simulink model "TRN_V3_2_CodeGen"  (R2022a)
settings: Solver=FixedStepAuto  StartTime=0.0  StopTime=300  FixedStep=0.04  RelTol=1e-3
PreLoadFcn:
  | load('BusStructureTRNsensor.mat');
  | addpath('C:/MAP');
InitFcn:
  | %load TRNDataBusPILS.mat
  | %addpath(genpath(cd))
  | 
  | %load('TPF_WHOLESIM_INPUT_SCENARIOS_AGCAS_N35_10E127_70.mat');
  | 
  | % Add DataBus Path
  | addpath(',,/');
  | addpath('../MAP/');
  | addpath('../MAP/MAP_DB');
  | addpath('../MAP/DVOF');
  | addpath(genpath(cd));
  | load('BusStructureTRN.mat');
undefined symbols (not defined in the file or in its folder): Altitude_INS, Latitude_INS, Longitude_INS, TRN, TRNlib
libraries: simulink_extras x23, aerolibconvert2 x6, sharedtransform x4, dspstat3 x2
(part 1 of 3)
settings Model: Creator=HSU  LastModifiedBy=ASCL
settings OptimizationCC: DefaultParameterBehavior=Inlined  UseDivisionForNetSlopeComputation=on  GainParamInheritBuiltInType=on  UseFloatMulNetSlope=on  PassReuseOutputArgsAs=Individual arguments  ZeroExternalMemoryAtStartup=off  ZeroInternalMemoryAtStartup=off  LifeSpan=Inf  OptimizeBlockOrder=speed  DifferentSizesBufferReuse=on  EfficientTunableParamExpr=on
settings DebuggingCC: ParameterTunabilityLossMsg=error  UnconnectedInputMsg=warning  UnconnectedOutputMsg=warning  UnconnectedLineMsg=warning  SFUnexpectedBacktrackingDiag=warning  SFNoUnconditionalDefaultTransitionDiag=warning
settings HardwareCC: ProdBitPerPointer=32  ProdBitPerSizeT=32  ProdBitPerPtrDiffT=32  ProdLargestAtomicInteger=Long  ProdLargestAtomicFloat=Double  ProdEndianess=BigEndian  ProdWordSize=32  ProdLongLongMode=on  ProdHWDeviceType=Freescale->MPC83xx
settings ModelReferenceCC: ModelReferenceNumInstancesAllowed=Single
settings SFSimCC: SimCustomHeaderCode="#include \"MAP.h\""  SimUserSources=MAP.c  SimUserLibraries=WS2_32.LIB  MATLABDynamicMemAlloc=off
settings RTWCC: SystemTargetFile=ert.tlc  GenCodeOnly=on  TemplateMakefile=ert_default_tmf  GenerateReport=on  RTWUseSimCustomCode=on  CustomHeaderCode="#include \"MAP.h\""  CustomSource=MAP.c  CustomLibrary=WS2_32.LIB  BuildConfiguration=Faster Runs  LaunchReport=on  GenerateCodeMetricsReport=on  DLArmComputeVersion=19.05
settings CodeAppCC: ForceParamTrailComments=on  IgnoreCustomStorageClasses=off  OperatorAnnotations=on  SimulinkDataObjDesc=on  SFDataObjDesc=on  MATLABFcnDesc=on  InsertBlockDesc=on  StateflowObjectComments=on  MATLABSourceComments=on  EnableCustomComments=on  ReqsInCode=on
settings ERTTargetCC: TargetLangStandard=C99 (ISO)  UtilityFuncGeneration=Shared location  GenerateSampleERTMain=on  SuppressErrorStatus=on  SupportAbsoluteTime=off  SupportNonFinite=off  SupportComplex=off  SupportVariableSizeSignals=on  ParenthesesLevel=Standards  CastingMode=Standards  InlinedParameterPlacement=NonHierarchical  ERTCustomFileTemplate=example_file_process.tlc  PreserveIfCondition=on  ConvertIfToSwitch=off  EnableSignedLeftShifts=off  EnableSignedRightShifts=off

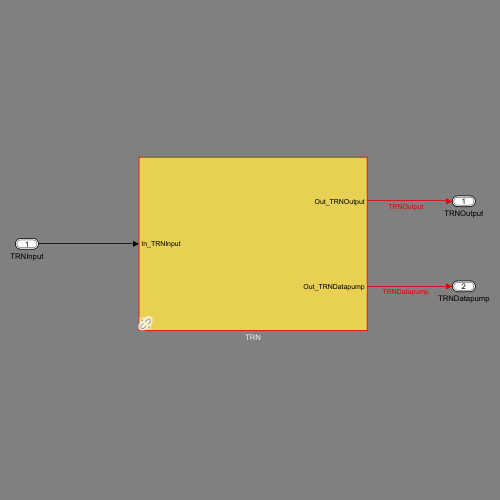
[thumbnail: Simulink's stored preview of the top-level diagram]
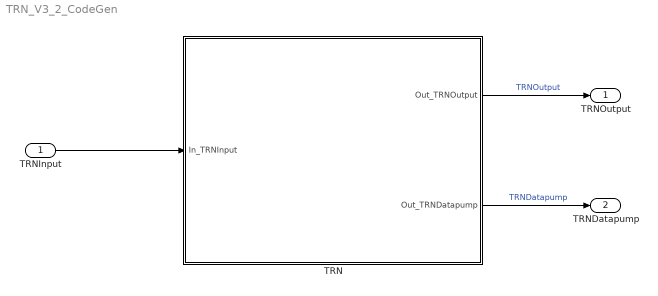
== system TRN_V3_2_CodeGen ==
  TRNInput : Inport  OutDataTypeStr=Bus: TRNInput  BusOutputAsStruct=on
  TRN : Subsystem  AncestorBlock=TRNlib/TRN
  TRNOutput : Outport  OutDataTypeStr=Bus: TRNOutput  VectorParamsAs1DForOutWhenUnconnected=off  BusOutputAsStruct=on
  TRNDatapump : Outport  Port=2  OutDataTypeStr=Bus: TRNDatapump  VectorParamsAs1DForOutWhenUnconnected=off  BusOutputAsStruct=on
  wires:
  TRN/2(Out_TRNDatapump) -> TRNDatapump/1  "TRNDatapump"
  TRN/1(Out_TRNOutput) -> TRNOutput/1  "TRNOutput"
  TRNInput/1 -> TRN/1(In_TRNInput)

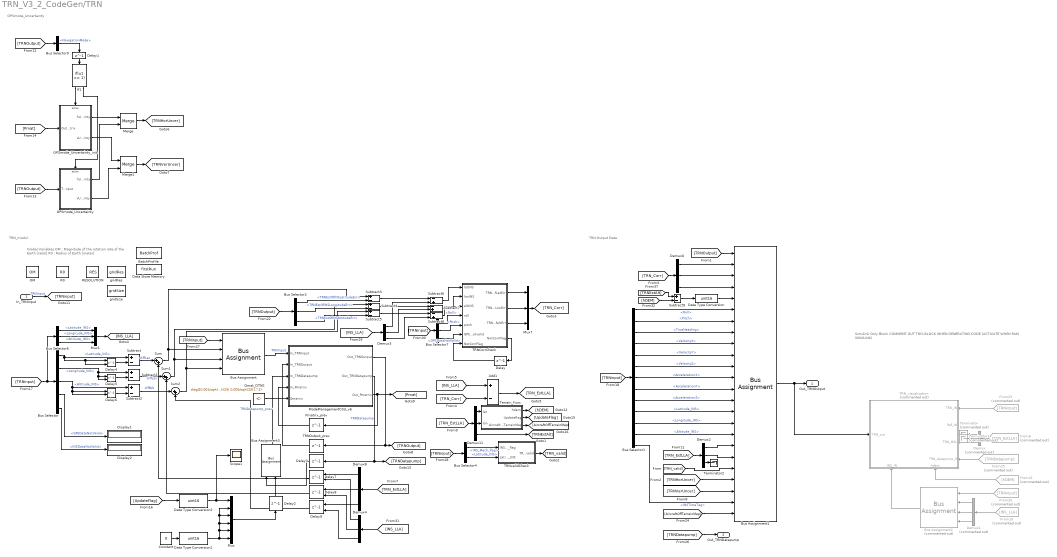
== system TRN_V3_2_CodeGen/TRN ==
  note: Global Variables
      | OM : Magnitude of the rotation rate of the Earth [rad/s]
      | R0 : Radius of Earth [meter]
  note: GPSmode_Uncertainty
  note: TRN Output Data
  note: TRN_modul
  note: Simulink Only Block
      | COMMENT OUT THIS BLOCK WHEN GENERATING CODE
      | (ACTIVATE WHEN RUN SIMULINK)
  In_TRNInput : Inport  OutDataTypeStr=Bus: TRNInput
  Add1 : Sum  Inputs=+-
  BatchProfile : DataStoreMemory  DataStoreName=BatchProf  ReadBeforeWriteMsg=warning  WriteAfterWriteMsg=warning  WriteAfterReadMsg=warning  ShowAdditionalParam=off  OutDataTypeStr=double  Dimensions=84200
  Bus Assignment : BusAssignment  AssignedSignals=Latitude_INS,Longitude_INS,Altitude_INS
  Bus Assignment1 : BusAssignment  AssignedSignals=TRNEstOfINSLatitudeErr,TRNEstOfINSLongitudeErr,TRNEstOfINSAltitudeErr,TRNEstHeightAGL,TRN_Roll,TRN_Pitch,TRN_Yaw,TRN_VelocityX,TRN_VelocityY,TRN_VelocityZ,TRN_AccelerationX,TRN_AccelerationY,TRN_AccelerationZ,Latitude_INS,Longitude_INS,Altitude_INS,TRNEstOfLatitude,TRNEstOfLongitude,TRN_valid,TRNHorUncertainty,TRNVerticalUncertainty,TRNTimeTag,AircraftOffTerrainMap
  Bus Assignment2 : BusAssignment  Commented=on  AssignedSignals=Latitude_INS,Longitude_INS,Altitude_INS
  Bus Assignment3 : BusAssignment  AssignedSignals=Result_Prev
  Bus Selector : BusSelector  OutputSignals=Latitude_INS,Longitude_INS,Altitude_INS,GPSDataNotValid,INSDataNotValid
  Bus Selector1 : BusSelector  OutputSignals=Roll,Pitch,TrueHeading,VelocityX,VelocityY,VelocityZ,AccelerationX,AccelerationY,AccelerationZ,Latitude_INS,Longitude_INS,Altitude_INS,INSTimeTag
  Bus Selector2 : BusSelector  OutputSignals=TRNEstOfINSLatitudeErr,TRNEstOfINSLongitudeErr,TRNEstOfINSAltitudeErr
  Bus Selector4 : BusSelector  OutputSignals=INS_Mech_flag,Latitude_INS
  Bus Selector6 : BusSelector  OutputSignals=Latitude_INS,Longitude_INS,Altitude_INS
  Bus Selector7 : BusSelector  OutputSignals=Roll,Pitch,GPSDataNotValid
  Bus Selector9 : BusSelector  OutputSignals=NavigationMode
  Constant : Constant  Value=0
  Data Store Memory : DataStoreMemory  DataStoreName=firstRun  ReadBeforeWriteMsg=warning  WriteAfterWriteMsg=warning  WriteAfterReadMsg=warning  InitialValue=logical(1)  VectorParams1D=off  ShowAdditionalParam=off  OutDataTypeStr=boolean
      settings: LockScale=on
  Data Type Conversion : DataTypeConversion  OutDataTypeStr=uint16  RndMeth=Nearest  SaturateOnIntegerOverflow=off
  Data Type Conversion1 : DataTypeConversion  OutDataTypeStr=uint16  SaturateOnIntegerOverflow=off  RndMeth=Floor
  Data Type Conversion2 : DataTypeConversion  OutDataTypeStr=uint16  SaturateOnIntegerOverflow=off  RndMeth=Floor
  Delay : Delay  DelayLength=1
  Delay1 : Delay  DelayLength=1  InitialCondition=1
  Delay2 : Delay  DelayLength=1  InitialCondition=0
  Delay3 : Delay  DelayLength=1  InitialCondition=0
  Delay4 : Delay  DelayLength=1  InitialConditionSource=Input port  InitialCondition=35.2*pi/180
      settings: InputPortMap=u0,p4
  Delay5 : Delay  DelayLength=1  InitialConditionSource=Input port  InitialCondition=35.2*pi/180
      settings: InputPortMap=u0,p4
  Delay6 : Delay  DelayLength=1  InitialConditionSource=Input port  InitialCondition=35.2*pi/180
      settings: InputPortMap=u0,p4
  Delay7 : Delay  DelayLength=1  InitialConditionSource=Input port  InitialCondition=0
      settings: InputPortMap=u0,p4
  Delay8 : Delay  DelayLength=1  InitialConditionSource=Input port  InitialCondition=0
      settings: InputPortMap=u0,p4
  Delay9 : Delay  DelayLength=1  InitialConditionSource=Input port  InitialCondition=0
      settings: InputPortMap=u0,p4
  Demux : Demux  Commented=on  Outputs=3
  Demux1 : Demux  Commented=on  Outputs=3
  Demux{2..4,6,8,11} (6 alike) : Demux  Outputs=3
  Display1 : Display
  Display2 : Display
  From10 : From  Commented=on  GotoTag=INS_LLA
  From20 : From  Commented=on  GotoTag=TRNinput
  From21 : From  Commented=on  GotoTag=hDEM
  From23 : From  Commented=on  GotoTag=TRNinput
  From25 : From  Commented=on  GotoTag=TRNDatapump
  From6 : From  Commented=on  GotoTag=TRN_EstLLA
  GPSmode_Uncertainty : Subsystem  TreatAsAtomicUnit=on
  GPSmode_Uncertainty_init : Subsystem  TreatAsAtomicUnit=on
  If1 : If  IfExpression=u1 == 1
  Merge : Merge
  Merge1 : Merge
  ModeManagementCSU_v6 : Stateflow chart  TreatAsAtomicUnit=on
  Mux : Mux  Inputs=6
  Mux1 : Mux  Inputs=3
  Mux7 : Mux  Inputs=3
  OM : DataStoreMemory  DataStoreName=OM  ReadBeforeWriteMsg=warning  WriteAfterWriteMsg=warning  WriteAfterReadMsg=warning  InitialValue=7.27e-5  ShowAdditionalParam=off
  Pmatrix_prev : Delay  DelayLength=1  InitialCondition="diag([0 0 0 0 0 0  10/6378000 10/6378000 13.3 0.0 0.0 0.0 0.00014 0.00014 0.00014 ].^2);"
  Qmat_DTNS : Constant  Value=diag([0.001/sqrt(25) 0.001/sqrt(25) 0.001/sqrt(25) 0.005/sqrt(25) 0.005/sqrt(25) 0.005/sqrt(25)].^2)
  R0 : DataStoreMemory  DataStoreName=R0  ReadBeforeWriteMsg=warning  WriteAfterWriteMsg=warning  WriteAfterReadMsg=warning  InitialValue=6378000  ShowAdditionalParam=off
  RESOLUTION : DataStoreMemory  DataStoreName=RES  ReadBeforeWriteMsg=warning  WriteAfterWriteMsg=warning  WriteAfterReadMsg=warning  InitialValue=3 * 0.000277777777777777 * 0.0174532925199433  ShowAdditionalParam=off  OutDataTypeStr=double
  Scope1 : Scope
  Subtract{,1..5,9} (7 alike) : Sum  Inputs=+-
  Subtract6 : Sum  Inputs=-+
  Subtract7 : Sum  Inputs=-+
  Subtract8 : Sum  Inputs=-+
  Sum : Sum  Inputs=|++
  Sum1 : Sum  Inputs=|++
  Sum2 : Sum  Inputs=|++
  TRNCorrCheck : MATLAB Function  TreatAsAtomicUnit=on
  TRNOutput_prev : Delay  DelayLength=1  InitialCondition=struct('NavigationMode', false);
  "TRN_visualization " : Subsystem  Commented=on
      settings: PortSchema="{\"entries\":[{\"content\":{\"sides\":[{\"content\":{\"connectorIds\":[\"In1\",\"In2\",\"In3\",\"In4\"]},\"type\":\"ConnectorPlacement.EquallySpacedRectSide\",\"uuid\":\"9b00cbc4-ca0d-429d-9536-38963fe71bc1\"},{\"content\":{\"connectorIds\":[\"In7\"],\"side\":\"RIGHT\"},\"type\":\"ConnectorPlacement.EquallySpacedRectSide\",\"uuid\":\"1db309fb-4b82-499a-a8dc-4a1ba85275fb\"},{\"content\":{\"connectorIds\":[\"In5\",\"In6\"],\"side\":\"TOP\"},\"type\":\"ConnectorPlacement.EquallySpacedRectSide\",\"uuid\":\"7e2d2316-30f0-423f-b46b-636ee0f4a770\"}]},\"type\":\"ConnectorPlacement.EquallySpacedConnector\",\"uuid\":\"aa6e905d-ed4c-45ad-a850-3c33939aad22\"}],\"packageUris\":[\"http://schema.mathworks.com/mf0/Connector/R2020b\"],\"version\":\"1.0\"}"
  TRNvalidCheck : MATLAB Function  TreatAsAtomicUnit=on
  Terminator : Terminator  Commented=on
  Terminator1 : Terminator  Commented=on
  Terminator2 : Terminator
  Terrain_Func : Subsystem
  gridRes : DataStoreMemory  DataStoreName=gridRes  ReadBeforeWriteMsg=warning  WriteAfterWriteMsg=warning  WriteAfterReadMsg=warning  InitialValue=0.1  ShowAdditionalParam=off  OutDataTypeStr=double
  gridSize : DataStoreMemory  DataStoreName=gridSize  ReadBeforeWriteMsg=warning  WriteAfterWriteMsg=warning  WriteAfterReadMsg=warning  InitialValue=20  ShowAdditionalParam=off  OutDataTypeStr=double
  Out_TRNOutput : Outport  OutDataTypeStr=Bus: TRNOutput  VectorParamsAs1DForOutWhenUnconnected=off
  Out_TRNDatapump : Outport  Port=2  OutDataTypeStr=Bus: TRNDatapump  VectorParamsAs1DForOutWhenUnconnected=off
  wires:
  Bus Selector2/2 -> Subtract4/2  "<TRNEstOfINSLongitudeErr>"
  Bus Selector2/1 -> Subtract3/2  "<TRNEstOfINSLatitudeErr>"
  Terrain_Func/1(hdem) -> [hDEM]
  Bus Selector4/1 -> TRNvalidCheck/1(INS_Mech_flag)  "<INS_Mech_flag>"
  Bus Selector4/2 -> TRNvalidCheck/2(Latitude_INS)  "<Latitude_INS>"
  [TRN_valid] -> Bus Assignment1/20
  TRNvalidCheck/1(TRN_valid) -> [TRN_valid]
  Bus Assignment/1 -> ModeManagementCSU_v6/1(In_TRNInput)  "TRNInput"
  Bus Selector/2 -> Delay5/1, Delay5/2, Subtract1/1  "<Longitude_INS>"
  Bus Selector1/3 -> Bus Assignment1/8  "<TrueHeading>"
  Bus Selector1/12 -> Bus Assignment1/17  "<Altitude_INS>"
  Bus Selector1/11 -> Bus Assignment1/16  "<Longitude_INS>"
  Bus Selector1/10 -> Bus Assignment1/15  "<Latitude_INS>"
  Bus Selector1/9 -> Bus Assignment1/14  "<AccelerationZ>"
  Bus Selector1/8 -> Bus Assignment1/13  "<AccelerationY>"
  Bus Selector1/7 -> Bus Assignment1/12  "<AccelerationX>"
  Bus Selector1/6 -> Bus Assignment1/11  "<VelocityZ>"
  Bus Selector1/5 -> Bus Assignment1/10  "<VelocityY>"
  Bus Selector1/4 -> Bus Assignment1/9  "<VelocityX>"
  Bus Selector1/2 -> Bus Assignment1/7  "<Pitch>"
  Bus Selector1/1 -> Bus Assignment1/6  "<Roll>"
  In_TRNInput/1 -> [TRNinput]  "TRNInput"
  ModeManagementCSU_v6/2(Out_TRNDatapump) -> Delay3/1, [TRNDatapump]  "TRNDatapump"
  TRNOutput_prev/1 -> ModeManagementCSU_v6/2(In_TRNOutput)
  Delay3/1 -> Bus Assignment3/1
  Bus Selector/3 -> Delay6/2, Delay6/1, Subtract2/1  "<Altitude_INS>"
  Bus Selector/1 -> Delay4/1, Delay4/2, Subtract/1  "<Latitude_INS>"
  Delay4/1 -> Subtract/2
  Delay5/1 -> Subtract1/2
  Delay6/1 -> Subtract2/2
  Sum/1 -> Subtract3/1, Bus Assignment/2
  Sum1/1 -> Subtract4/1, Bus Assignment/3
  Sum2/1 -> Subtract5/1, Bus Assignment/4
  Subtract/1 -> Sum/1  "diffLat"
  Subtract1/1 -> Sum1/1  "diffLon"
  Subtract4/1 -> Subtract7/1
  Subtract2/1 -> Sum2/1  "diffAlt"
  Delay7/1 -> Sum/2
  Delay8/1 -> Sum1/2
  Delay9/1 -> Sum2/2
  Bus Assignment1/1 -> "TRN_visualization "/7(TRN_out), Out_TRNOutput/1
  Subtract9/1 -> Data Type Conversion/1
  Data Type Conversion/1 -> Bus Assignment1/5
  Subtract6/1 -> TRNCorrCheck/1(latINS)
  Subtract7/1 -> TRNCorrCheck/2(lonINS)
  Subtract8/1 -> TRNCorrCheck/3(altINS)
  TRNCorrCheck/3(TRNEstOfaltErr) -> Mux7/3
  [TRN_Corr] -> Demux6/1
  Demux6/1 -> Bus Assignment1/2
  Demux6/2 -> Bus Assignment1/3
  Demux6/3 -> Bus Assignment1/4
  TRNCorrCheck/1(TRNEstOfLatErr) -> Mux7/1
  TRNCorrCheck/2(TRNEstOfLonErr) -> Mux7/2
  Subtract5/1 -> Subtract8/1
  Subtract3/1 -> Subtract6/1
  [TRN_EstLLA] -> Demux8/1
  Demux8/1 -> Delay7/1
  Demux8/2 -> Delay8/1
  Demux8/3 -> Delay9/1
  Mux1/1 -> [INS_LLA]
  Bus Selector6/2 -> Mux1/2  "<Longitude_INS>"
  Bus Selector6/3 -> Mux1/3  "<Altitude_INS>"
  [INS_LLA] -> Add1/1
  Add1/1 -> [TRN_EstLLA]
  Demux11/1 -> Terrain_Func/1(lat)
  Demux11/2 -> Terrain_Func/2(lon)
  TRNCorrCheck/4(NotCorrFlag) -> Delay/1
  Delay/1 -> TRNCorrCheck/7("NotCorrFlag ")
  [TRN_EstLLA] -> Demux11/1
  Qmat_DTNS/1 -> ModeManagementCSU_v6/5(Qmatrix)
  ModeManagementCSU_v6/3(Out_Pmatrix) -> Pmatrix_prev/1, [Pmat]
  Bus Selector/4 -> Display1/1  "<GPSDataNotValid>"
  Mux7/1 -> [TRN_Corr]
  If1/1 -> GPSmode_Uncertainty_init/Action
  If1/2 -> GPSmode_Uncertainty/Action
  GPSmode_Uncertainty_init/1(hUncertainty) -> Merge/1
  GPSmode_Uncertainty/1(hUncertainty) -> Merge/2
  GPSmode_Uncertainty_init/2(vUncertainty) -> Merge1/1
  GPSmode_Uncertainty/2(vUncertainty) -> Merge1/2
  Bus Selector9/1 -> Delay1/1  "<NavigationMode>"
  Merge/1 -> [TRNHorUncer]
  Merge1/1 -> [TRNVerUncer]
  [TRNVerUncer] -> Bus Assignment1/22
  Demux2/1 -> Bus Assignment1/18
  Demux2/2 -> Bus Assignment1/19
  [TRN_EstLLA] -> Demux2/1
  [TRNOutput] -> Bus Selector9/1
  [TRNOutput] -> GPSmode_Uncertainty/1(TRNOutput)
  [Pmat] -> GPSmode_Uncertainty_init/1(Out_Pmatrix)
  [TRNinput] -> Bus Selector6/1, Bus Selector/1
  [TRNinput] -> Bus Selector1/1
  [TRNDatapump] -> Out_TRNDatapump/1
  [TRNinput] -> Bus Assignment/1
  Delay1/1 -> If1/1
  [TRNOutput] -> Bus Assignment1/1
  Bus Selector2/3 -> Subtract5/2  "<TRNEstOfINSAltitudeErr>"
  [TRNOutput] -> Bus Selector2/1
  [INS_LLA] -> Demux3/1
  Demux3/1 -> Subtract6/2
  Demux3/2 -> Subtract7/2
  Demux3/3 -> Subtract8/2
  [TRNinput] -> Bus Selector7/1
  Bus Selector7/1 -> TRNCorrCheck/4(roll)  "<Roll>"
  Bus Selector7/2 -> TRNCorrCheck/5(pitch)  "<Pitch>"
  Bus Selector6/1 -> Mux1/1  "<Latitude_INS>"
  [INS_LLA] -> Demux4/1
  Demux4/1 -> Delay7/2
  Demux4/2 -> Delay8/2
  Demux4/3 -> Delay9/2
  Bus Selector7/3 -> TRNCorrCheck/6(GPSDataNotvalid)  "<GPSDataNotValid>"
  [hDEM] -> Subtract9/2
  Demux11/3 -> [TRNEstAlt]
  [TRNEstAlt] -> Subtract9/1
  Bus Selector1/13 -> Bus Assignment1/23  "<INSTimeTag>"
  Bus Assignment2/1 -> "TRN_visualization "/6(INS_IN)
  Demux1/1 -> Bus Assignment2/2
  From20/1 -> Bus Assignment2/1
  From10/1 -> Demux1/1
  From6/1 -> Demux/1
  From23/1 -> "TRN_visualization "/4(TRN_IN)
  Demux/3 -> "TRN_visualization "/2(TRN_MSL)
  From21/1 -> "TRN_visualization "/5(hdem)
  Demux1/3 -> Bus Assignment2/4
  From25/1 -> "TRN_visualization "/1(TRN_datapump_IN)
  Demux1/2 -> Bus Assignment2/3
  Bus Assignment3/1 -> ModeManagementCSU_v6/3(In_TRNDatapump)  "TRNDatapump_prev"
  [TRNinput] -> Bus Selector4/1
  ModeManagementCSU_v6/1(Out_TRNOutput) -> TRNOutput_prev/1, [TRNOutput]
  [TRNHorUncer] -> Bus Assignment1/21
  Bus Selector/5 -> Display2/1  "<INSDataNotValid>"
  [TRN_Corr] -> Add1/2
  Mux/1 -> Delay2/1
  Terrain_Func/2(Updateflag) -> [UpdateFlag]
  Constant/1 -> Data Type Conversion1/1
  Terrain_Func/3(AircraftOffTerrainMap) -> [AircraftOffTerrainMap]
  [AircraftOffTerrainMap] -> Bus Assignment1/24
  Data Type Conversion1/1 -> Mux/2, Mux/3, Mux/4, Mux/5, Mux/6
  [UpdateFlag] -> Data Type Conversion2/1
  Data Type Conversion2/1 -> Scope1/1, Mux/1
  Delay2/1 -> Bus Assignment3/2
  Pmatrix_prev/1 -> ModeManagementCSU_v6/4(In_Pmatrix)
  Demux/1 -> Terminator/1
  Demux/2 -> Terminator1/1
  Demux2/3 -> Terminator2/1

== system TRN_V3_2_CodeGen/TRN/GPSmode_Uncertainty ==
  TRNOutput : Inport
  Action Port : ActionPort  ActionPortLabel=else
  Bus Selector : BusSelector  OutputSignals=TRNHorUncertainty,TRNVerticalUncertainty
  Scope : Scope  NumInputPorts=2
  hUncertainty : Outport
  vUncertainty : Outport  Port=2
  wires:
  TRNOutput/1 -> Bus Selector/1
  Bus Selector/1 -> Scope/1, hUncertainty/1  "<TRNHorUncertainty>"
  Bus Selector/2 -> vUncertainty/1, Scope/2  "<TRNVerticalUncertainty>"

== system TRN_V3_2_CodeGen/TRN/GPSmode_Uncertainty_init ==
  Out_Pmatrix : Inport
  Action Port : ActionPort  ActionPortLabel=if(u1 == 1)
  Uncertainty_init : MATLAB Function  TreatAsAtomicUnit=on
  hUncertainty : Outport
  vUncertainty : Outport  Port=2
  wires:
  Out_Pmatrix/1 -> Uncertainty_init/1(P)
  Uncertainty_init/1(hUncertainty) -> hUncertainty/1
  Uncertainty_init/2(vUncertainty) -> vUncertainty/1

== system TRN_V3_2_CodeGen/TRN/ModeManagementCSU_v6/CollectProfile ==
  In_TRNDatapump : Inport  OutDataTypeStr=Bus: TRNDatapump  PortDimensions=1
  f : TriggerPort  TriggerType=function-call  VariantControl=Variant
      settings: CopyFcn=Stateflow.SLINSF.SimulinkMan.removeBlockPreDeleteFcn  PreDeleteFcn=Stateflow.SLINSF.SimulinkMan.unsafePredeleteFcn
  Bus Selector1 : BusSelector  OutputSignals=profileCnt
  CollectProfile function : MATLAB Function  TreatAsAtomicUnit=on
  Data Store Read : DataStoreRead  DataStoreName=gridRes  IndexOptions=Index vector (dialog)  Indices=1  OutputSizes=1
  Data Store Read1 : DataStoreRead  DataStoreName=RES  IndexOptions=Index vector (dialog)  Indices=1  OutputSizes=1
  Data Store Read2 : DataStoreRead  DataStoreName=gridSize  IndexOptions=Index vector (dialog)  Indices=1  OutputSizes=1
  Data Store Read3 : DataStoreRead  DataStoreName=BatchProf  IndexOptions=Index vector (dialog)  Indices=1  OutputSizes=1
  Data Store Write : DataStoreWrite  DataStoreName=BatchProf  IndexOptions=Index vector (dialog)  Indices=1  OutputSizes=1
  Scope : Scope
  wires:
  CollectProfile function/2(batchProfile) -> Data Store Write/1
  Data Store Read2/1 -> CollectProfile function/3(gridSize)
  Data Store Read1/1 -> CollectProfile function/4(resolution)
  In_TRNDatapump/1 -> Bus Selector1/1
  Bus Selector1/1 -> CollectProfile function/2(profileCnt)  "<profileCnt>"
  CollectProfile function/1(hDEM) -> Scope/1
  Data Store Read/1 -> CollectProfile function/5(gridRes)
  Data Store Read3/1 -> CollectProfile function/1("batchProfile ")

== system TRN_V3_2_CodeGen/TRN/ModeManagementCSU_v6/CorrelationAnalysis ==
  In_TRNDatapump : Inport  OutDataTypeStr=Bus: TRNDatapump  PortDimensions=1
  f : TriggerPort  TriggerType=function-call  VariantControl=Variant
      settings: CopyFcn=Stateflow.SLINSF.SimulinkMan.removeBlockPreDeleteFcn  PreDeleteFcn=Stateflow.SLINSF.SimulinkMan.unsafePredeleteFcn
  Bus Selector1 : BusSelector  OutputSignals=profileCnt
  CorrelationAnalysis function : MATLAB Function  TreatAsAtomicUnit=on
  Data Store Read : DataStoreRead  DataStoreName=BatchProf  IndexOptions=Index vector (dialog)  Indices=1  OutputSizes=1
  Data Store Read1 : DataStoreRead  DataStoreName=RES  IndexOptions=Index vector (dialog)  Indices=1  OutputSizes=1
  Data Store Read2 : DataStoreRead  DataStoreName=gridRes  IndexOptions=Index vector (dialog)  Indices=1  OutputSizes=1
  Data Store Read3 : DataStoreRead  DataStoreName=gridSize  IndexOptions=Index vector (dialog)  Indices=1  OutputSizes=1
  Scope : Scope  NumInputPorts=2
  Scope1 : Scope
  posUpdate : Outport  VectorParamsAs1DForOutWhenUnconnected=off
  MAD : Outport  Port=2  OutDataTypeStr=single  VectorParamsAs1DForOutWhenUnconnected=off
  residual : Outport  Port=3
  wires:
  CorrelationAnalysis function/2(MAD) -> Scope/1, MAD/1
  CorrelationAnalysis function/1(posUpdate) -> posUpdate/1
  CorrelationAnalysis function/3(residual) -> Scope/2, residual/1
  Data Store Read1/1 -> CorrelationAnalysis function/4(resolution)
  In_TRNDatapump/1 -> Bus Selector1/1
  Bus Selector1/1 -> Scope1/1, CorrelationAnalysis function/2(profileCnt)  "<profileCnt>"
  Data Store Read2/1 -> CorrelationAnalysis function/5(gridRes)
  Data Store Read3/1 -> CorrelationAnalysis function/3(gridSize)
  Data Store Read/1 -> CorrelationAnalysis function/1(batchProfile)

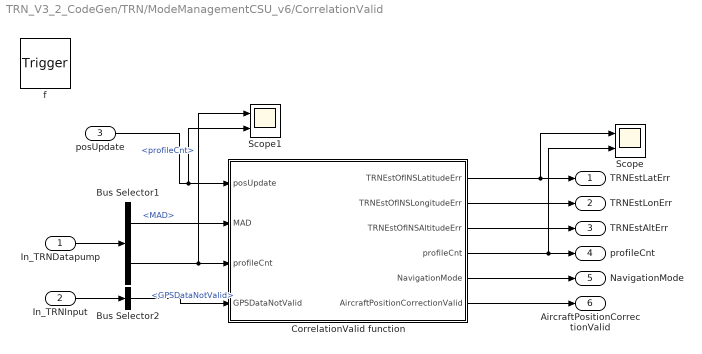
== system TRN_V3_2_CodeGen/TRN/ModeManagementCSU_v6/CorrelationValid ==
  In_TRNDatapump : Inport  OutDataTypeStr=Bus: TRNDatapump  PortDimensions=1
  In_TRNInput : Inport  Port=2  OutDataTypeStr=Bus: TRNInput  PortDimensions=1
  posUpdate : Inport  Port=3  OutDataTypeStr=double  PortDimensions=2
  f : TriggerPort  TriggerType=function-call  VariantControl=Variant
      settings: CopyFcn=Stateflow.SLINSF.SimulinkMan.removeBlockPreDeleteFcn  PreDeleteFcn=Stateflow.SLINSF.SimulinkMan.unsafePredeleteFcn
  Bus Selector1 : BusSelector  OutputSignals=MAD,profileCnt
  Bus Selector2 : BusSelector  OutputSignals=GPSDataNotValid
  CorrelationValid function : MATLAB Function  TreatAsAtomicUnit=on
  Scope : Scope  NumInputPorts=2
  Scope1 : Scope  NumInputPorts=2
  TRNEstLatErr : Outport  VectorParamsAs1DForOutWhenUnconnected=off
  TRNEstLonErr : Outport  Port=2  VectorParamsAs1DForOutWhenUnconnected=off
  TRNEstAltErr : Outport  Port=3
  profileCnt : Outport  Port=4  OutDataTypeStr=uint32
  NavigationMode : Outport  Port=5  OutDataTypeStr=boolean
  AircraftPositionCorrectionValid : Outport  Port=6
  wires:
  In_TRNDatapump/1 -> Bus Selector1/1
  Bus Selector1/2 -> Scope1/1, CorrelationValid function/3("profileCnt ")  "<profileCnt>"
  Bus Selector2/1 -> CorrelationValid function/4(GPSDataNotValid)  "<GPSDataNotValid>"
  In_TRNInput/1 -> Bus Selector2/1
  Bus Selector1/1 -> CorrelationValid function/2(MAD)  "<MAD>"
  CorrelationValid function/1(TRNEstOfINSLatitudeErr) -> Scope/1, TRNEstLatErr/1
  CorrelationValid function/2(TRNEstOfINSLongitudeErr) -> TRNEstLonErr/1
  CorrelationValid function/3(TRNEstOfINSAltitudeErr) -> TRNEstAltErr/1
  CorrelationValid function/4(profileCnt) -> Scope/2, profileCnt/1
  CorrelationValid function/5(NavigationMode) -> NavigationMode/1
  CorrelationValid function/6(AircraftPositionCorrectionValid) -> AircraftPositionCorrectionValid/1
  posUpdate/1 -> Scope1/2, CorrelationValid function/1(posUpdate)

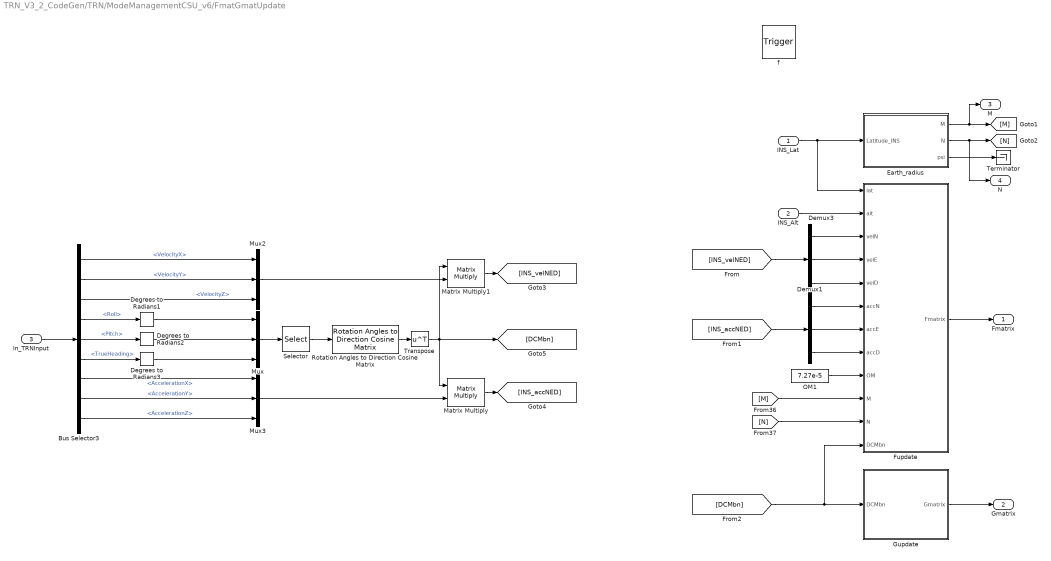
== system TRN_V3_2_CodeGen/TRN/ModeManagementCSU_v6/FmatGmatUpdate ==
  INS_Lat : Inport  OutDataTypeStr=double  PortDimensions=1
  INS_Alt : Inport  Port=2  OutDataTypeStr=double  PortDimensions=1
  In_TRNInput : Inport  Port=3  OutDataTypeStr=Bus: TRNInput  PortDimensions=1
  f : TriggerPort  TriggerType=function-call  VariantControl=Variant
      settings: CopyFcn=Stateflow.SLINSF.SimulinkMan.removeBlockPreDeleteFcn  PreDeleteFcn=Stateflow.SLINSF.SimulinkMan.unsafePredeleteFcn
  Bus Selector3 : BusSelector  OutputSignals=VelocityX,VelocityY,VelocityZ,Roll,Pitch,TrueHeading,AccelerationX,AccelerationY,AccelerationZ
  Degrees to Radians1 : simulink_extras/Transformations/Degrees to Radians
  Degrees to Radians2 : simulink_extras/Transformations/Degrees to Radians
  Degrees to Radians3 : simulink_extras/Transformations/Degrees to Radians
  Demux1 : Demux  Outputs=3
  Demux3 : Demux  Outputs=3
  Earth_radius : MATLAB Function  TreatAsAtomicUnit=on
  Fupdate : MATLAB Function  TreatAsAtomicUnit=on
  Gupdate : MATLAB Function  TreatAsAtomicUnit=on
  Matrix Multiply : Product  Multiplication=Matrix(*)
  Matrix Multiply1 : Product  Multiplication=Matrix(*)
  Mux : Mux  Inputs=3
  Mux2 : Mux  Inputs=3
  Mux3 : Mux  Inputs=3
  OM1 : Constant  Value=7.27e-5
  Rotation Angles to Direction Cosine Matrix : sharedtransform/Rotation Angles to Direction Cosine Matrix  rotationOrder=ZYX  aMode=aMode
      settings: SourceProductBaseCode=AE,PW,DR,MT,VE
  Selector : Selector  InputPortWidth=3  IndexOptions=Index vector (dialog)  Indices=[3 2 1]  OutputSizes=1
  Terminator : Terminator
  Transpose : Math  Operator=transpose  SignedPower=on
  Fmatrix : Outport
  Gmatrix : Outport  Port=2
  M : Outport  Port=3
  N : Outport  Port=4
  wires:
  Earth_radius/1(M) -> M/1, [M]
  Earth_radius/2(N) -> N/1, [N]
  Earth_radius/3(psi) -> Terminator/1
  Gupdate/1(Gmatrix) -> Gmatrix/1
  Fupdate/1(Fmatrix) -> Fmatrix/1
  [INS_velNED] -> Demux3/1
  Demux1/2 -> Fupdate/7(accE)
  [M] -> Fupdate/10(M)
  OM1/1 -> Fupdate/9(OM)
  Demux3/2 -> Fupdate/4(velE)
  Demux3/1 -> Fupdate/3(velN)
  Demux3/3 -> Fupdate/5(velD)
  [DCMbn] -> Gupdate/1(DCMbn), Fupdate/12(DCMbn)
  Demux1/1 -> Fupdate/6(accN)
  [INS_accNED] -> Demux1/1
  Demux1/3 -> Fupdate/8(accD)
  [N] -> Fupdate/11(N)
  Bus Selector3/3 -> Mux2/3  "<VelocityZ>"
  Bus Selector3/6 -> Degrees to Radians3/1  "<TrueHeading>"
  Bus Selector3/5 -> Degrees to Radians2/1  "<Pitch>"
  Bus Selector3/4 -> Degrees to Radians1/1  "<Roll>"
  Bus Selector3/1 -> Mux2/1  "<VelocityX>"
  Mux2/1 -> Matrix Multiply1/2
  Bus Selector3/2 -> Mux2/2  "<VelocityY>"
  Mux/1 -> Selector/1
  Matrix Multiply1/1 -> [INS_velNED]
  Degrees to Radians2/1 -> Mux/2
  Rotation Angles to Direction Cosine Matrix/1 -> Transpose/1
  Degrees to Radians1/1 -> Mux/1
  In_TRNInput/1 -> Bus Selector3/1
  Selector/1 -> Rotation Angles to Direction Cosine Matrix/1
  Degrees to Radians3/1 -> Mux/3
  Bus Selector3/7 -> Mux3/1  "<AccelerationX>"
  Bus Selector3/9 -> Mux3/3  "<AccelerationZ>"
  Bus Selector3/8 -> Mux3/2  "<AccelerationY>"
  Transpose/1 -> [DCMbn], Matrix Multiply1/1, Matrix Multiply/1
  Mux3/1 -> Matrix Multiply/2
  Matrix Multiply/1 -> [INS_accNED]
  INS_Lat/1 -> Fupdate/1(lat), Earth_radius/1(Latitude_INS)
  INS_Alt/1 -> Fupdate/2(alt)

== system TRN_V3_2_CodeGen/TRN/ModeManagementCSU_v6/SetProfile ==
  In_TRNDatapump : Inport  OutDataTypeStr=Bus: TRNDatapump  PortDimensions=1
  In_TRNInput : Inport  Port=2  OutDataTypeStr=Bus: TRNInput  PortDimensions=1
  f : TriggerPort  TriggerType=function-call  VariantControl=Variant
      settings: CopyFcn=Stateflow.SLINSF.SimulinkMan.removeBlockPreDeleteFcn  PreDeleteFcn=Stateflow.SLINSF.SimulinkMan.unsafePredeleteFcn
  Bus Selector1 : BusSelector  OutputSignals=profileCnt
  ConvertTRNInput : Subsystem  TreatAsAtomicUnit=on
  Data Store Read : DataStoreRead  DataStoreName=BatchProf  IndexOptions=Index vector (dialog)  Indices=1  OutputSizes=1
  Data Store Read1 : DataStoreRead  DataStoreName=gridSize  IndexOptions=Index vector (dialog)  Indices=1  OutputSizes=1
  Data Store Write : DataStoreWrite  DataStoreName=BatchProf  IndexOptions=Index vector (dialog)  Indices=1  OutputSizes=1
  SetProfile function : MATLAB Function  TreatAsAtomicUnit=on
  wires:
  Bus Selector1/1 -> SetProfile function/9(profileCnt)  "<profileCnt>"
  In_TRNDatapump/1 -> Bus Selector1/1
  In_TRNInput/1 -> ConvertTRNInput/1(TRNInput)
  ConvertTRNInput/1(latINS) -> SetProfile function/1(latINS)
  ConvertTRNInput/2(lonINS) -> SetProfile function/2(lonINS)
  ConvertTRNInput/3(altINS) -> SetProfile function/3(altINS)
  ConvertTRNInput/4(altRALT) -> SetProfile function/4(RALT)
  ConvertTRNInput/5(latGPS) -> SetProfile function/5(latGPS)
  ConvertTRNInput/6(lonGPS) -> SetProfile function/6(lonGPS)
  ConvertTRNInput/7(altGPS) -> SetProfile function/7(altGPS)
  ConvertTRNInput/8(flagGPS) -> SetProfile function/8(flagGPS)
  Data Store Read/1 -> SetProfile function/10("batchProfile ")
  SetProfile function/1(batchProfile) -> Data Store Write/1
  Data Store Read1/1 -> SetProfile function/11(gridSize)

== system TRN_V3_2_CodeGen/TRN/ModeManagementCSU_v6/StoreProfile ==
  In_TRNInput : Inport  OutDataTypeStr=Bus: TRNInput  PortDimensions=1
  In_TRNDatapump : Inport  Port=2  OutDataTypeStr=Bus: TRNDatapump  PortDimensions=1
  f : TriggerPort  TriggerType=function-call  VariantControl=Variant
      settings: CopyFcn=Stateflow.SLINSF.SimulinkMan.removeBlockPreDeleteFcn  PreDeleteFcn=Stateflow.SLINSF.SimulinkMan.unsafePredeleteFcn
  Bus Selector1 : BusSelector  OutputSignals=profileCnt
  Bus Selector2 : BusSelector  OutputSignals=INSDataNotValid
  Data Store Read : DataStoreRead  DataStoreName=BatchProf  IndexOptions=Index vector (dialog)  Indices=1  OutputSizes=1
  Data Store Read1 : DataStoreRead  DataStoreName=gridSize  IndexOptions=Index vector (dialog)  Indices=1  OutputSizes=1
  Data Store Write : DataStoreWrite  DataStoreName=BatchProf  IndexOptions=Index vector (dialog)  Indices=1  OutputSizes=1
  Scope : Scope
  SetProfile function : MATLAB Function  TreatAsAtomicUnit=on
  profileCnt : Outport  PortDimensions=1  VectorParamsAs1DForOutWhenUnconnected=off
  wires:
  In_TRNInput/1 -> Bus Selector2/1
  Data Store Read/1 -> SetProfile function/1("batchProfile ")
  Bus Selector1/1 -> SetProfile function/2("profileCnt ")  "<profileCnt>"
  In_TRNDatapump/1 -> Bus Selector1/1
  SetProfile function/1(batchProfile) -> Data Store Write/1
  SetProfile function/2(profileCnt) -> profileCnt/1, Scope/1
  Data Store Read1/1 -> SetProfile function/3(gridSize)
  Bus Selector2/1 -> SetProfile function/4(flagINS)  "<INSDataNotValid>"

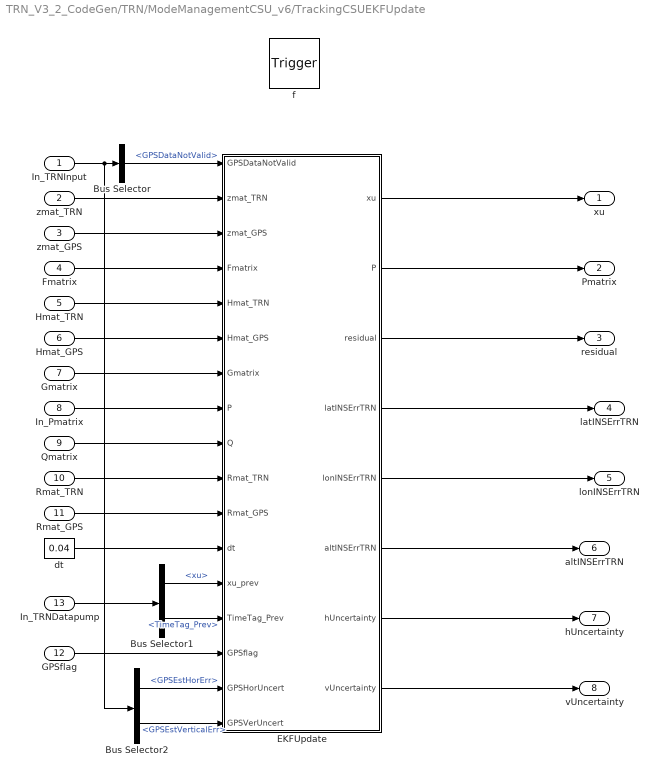
== system TRN_V3_2_CodeGen/TRN/ModeManagementCSU_v6/TrackingCSUEKFUpdate ==
  In_TRNInput : Inport  OutDataTypeStr=Bus: TRNInput  PortDimensions=1
  zmat_TRN : Inport  Port=2  OutDataTypeStr=double  PortDimensions=1
  zmat_GPS : Inport  Port=3  OutDataTypeStr=double  PortDimensions=[6 1]
  Fmatrix : Inport  Port=4  OutDataTypeStr=double  PortDimensions=[15 15]
  Hmat_TRN : Inport  Port=5  OutDataTypeStr=double  PortDimensions=[1 15]
  Hmat_GPS : Inport  Port=6  OutDataTypeStr=double  PortDimensions=[6 15]
  Gmatrix : Inport  Port=7  OutDataTypeStr=double  PortDimensions=[15 6]
  In_Pmatrix : Inport  Port=8  OutDataTypeStr=double  PortDimensions=[15 15]
  Qmatrix : Inport  Port=9  OutDataTypeStr=double  PortDimensions=[6 6]
  Rmat_TRN : Inport  Port=10  OutDataTypeStr=double  PortDimensions=1
  Rmat_GPS : Inport  Port=11  OutDataTypeStr=double  PortDimensions=[6 6]
  GPSflag : Inport  Port=12  OutDataTypeStr=uint32  PortDimensions=1
  In_TRNDatapump : Inport  Port=13  OutDataTypeStr=Bus: TRNDatapump  PortDimensions=1
  f : TriggerPort  TriggerType=function-call  VariantControl=Variant
      settings: CopyFcn=Stateflow.SLINSF.SimulinkMan.removeBlockPreDeleteFcn  PreDeleteFcn=Stateflow.SLINSF.SimulinkMan.unsafePredeleteFcn
  Bus Selector : BusSelector  OutputSignals=GPSDataNotValid
  Bus Selector1 : BusSelector  OutputSignals=xu,TimeTag_Prev
  Bus Selector2 : BusSelector  OutputSignals=GPSEstHorErr,GPSEstVerticalErr
  EKFUpdate : MATLAB Function  TreatAsAtomicUnit=on
  dt : Constant  Value=0.04  OutDataTypeStr=double
  xu : Outport
  Pmatrix : Outport  Port=2
  residual : Outport  Port=3
  latINSErrTRN : Outport  Port=4
  lonINSErrTRN : Outport  Port=5
  altINSErrTRN : Outport  Port=6
  hUncertainty : Outport  Port=7
  vUncertainty : Outport  Port=8
  wires:
  EKFUpdate/7(hUncertainty) -> hUncertainty/1
  Rmat_GPS/1 -> EKFUpdate/11(Rmat_GPS)
  Rmat_TRN/1 -> EKFUpdate/10(Rmat_TRN)
  Gmatrix/1 -> EKFUpdate/7(Gmatrix)
  EKFUpdate/8(vUncertainty) -> vUncertainty/1
  Hmat_TRN/1 -> EKFUpdate/5(Hmat_TRN)
  EKFUpdate/1(xu) -> xu/1
  EKFUpdate/5(lonINSErrTRN) -> lonINSErrTRN/1
  Hmat_GPS/1 -> EKFUpdate/6(Hmat_GPS)
  zmat_TRN/1 -> EKFUpdate/2(zmat_TRN)
  EKFUpdate/6(altINSErrTRN) -> altINSErrTRN/1
  zmat_GPS/1 -> EKFUpdate/3(zmat_GPS)
  EKFUpdate/2(P) -> Pmatrix/1
  EKFUpdate/3(residual) -> residual/1
  In_Pmatrix/1 -> EKFUpdate/8("P ")
  EKFUpdate/4(latINSErrTRN) -> latINSErrTRN/1
  Fmatrix/1 -> EKFUpdate/4(Fmatrix)
  GPSflag/1 -> EKFUpdate/15(GPSflag)
  dt/1 -> EKFUpdate/12(dt)
  Qmatrix/1 -> EKFUpdate/9(Q)
  Bus Selector1/1 -> EKFUpdate/13(xu_prev)  "<xu>"
  In_TRNDatapump/1 -> Bus Selector1/1
  In_TRNInput/1 -> Bus Selector2/1, Bus Selector/1
  Bus Selector/1 -> EKFUpdate/1(GPSDataNotValid)  "<GPSDataNotValid>"
  Bus Selector1/2 -> EKFUpdate/14(TimeTag_Prev)  "<TimeTag_Prev>"
  Bus Selector2/1 -> EKFUpdate/16(GPSHorUncert)  "<GPSEstHorErr>"
  Bus Selector2/2 -> EKFUpdate/17(GPSVerUncert)  "<GPSEstVerticalErr>"

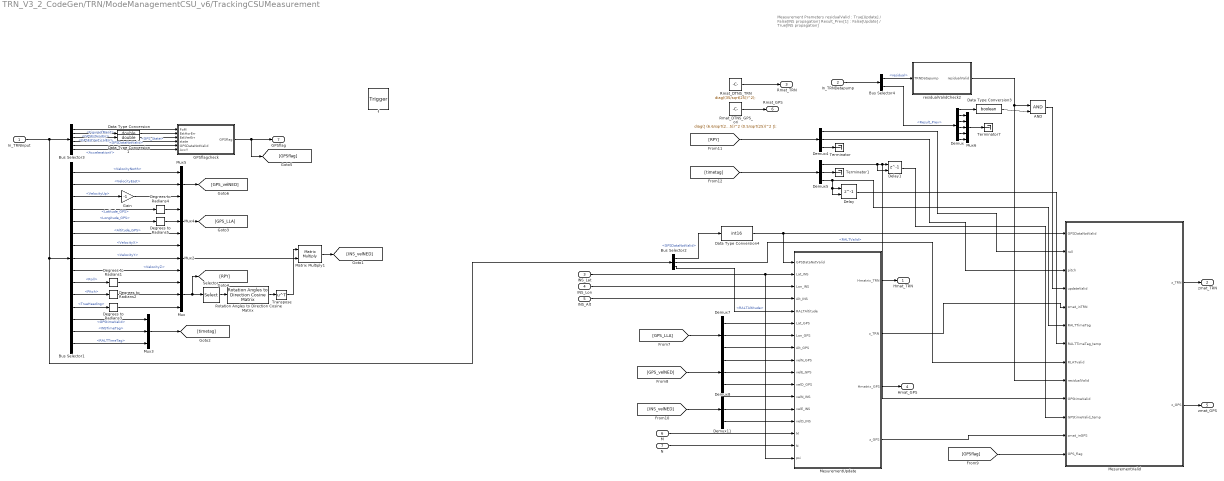
== system TRN_V3_2_CodeGen/TRN/ModeManagementCSU_v6/TrackingCSUMeasurement ==
  note: Measurement Prameters
      | residualValid : True[Update] / False[INS propagation]
      | Result_Prev[1] : False[Update] / True[INS propagation]
  In_TRNInput : Inport  OutDataTypeStr=Bus: TRNInput  PortDimensions=1
  In_TRNDatapump : Inport  Port=2  OutDataTypeStr=Bus: TRNDatapump  PortDimensions=1
  INS_Lat : Inport  Port=3  OutDataTypeStr=double  PortDimensions=1
  INS_Lon : Inport  Port=4  OutDataTypeStr=double  PortDimensions=1
  INS_Alt : Inport  Port=5  OutDataTypeStr=double  PortDimensions=1
  M : Inport  Port=6  OutDataTypeStr=double  PortDimensions=1
  N : Inport  Port=7  OutDataTypeStr=double  PortDimensions=1
  f : TriggerPort  TriggerType=function-call  VariantControl=Variant
      settings: CopyFcn=Stateflow.SLINSF.SimulinkMan.removeBlockPreDeleteFcn  PreDeleteFcn=Stateflow.SLINSF.SimulinkMan.unsafePredeleteFcn
  AND : Logic  IconShape=distinctive  AllPortsSameDT=off  OutDataTypeStr=boolean
  Bus Selector1 : BusSelector  OutputSignals=VelocityNorth,VelocityEast,VelocityUp,Latitude_GPS,Longitude_GPS,Altitude_GPS,VelocityX,VelocityY,VelocityZ,Roll,Pitch,TrueHeading,GPStimeValid,INSTimeTag,RALTTimeTag
  Bus Selector2 : BusSelector  OutputSignals=GPSDataNotValid,RALTValid,RALTAltitude
  Bus Selector3 : BusSelector  OutputSignals=FigureofMerit,GPSEstHorErr,GPSEstVerticalErr,GPS_State,GPSDataNotValid,AccelerationY
  Bus Selector4 : BusSelector  OutputSignals=residual,Result_Prev
  Data Type Conversion : DataTypeConversion  OutDataTypeStr=double  SaturateOnIntegerOverflow=off  RndMeth=Floor
  Data Type Conversion1 : DataTypeConversion  OutDataTypeStr=double  SaturateOnIntegerOverflow=off  RndMeth=Floor
  Data Type Conversion3 : DataTypeConversion  OutDataTypeStr=boolean  SaturateOnIntegerOverflow=off  RndMeth=Floor
  Data Type Conversion4 : DataTypeConversion  OutDataTypeStr=int16  SaturateOnIntegerOverflow=off  RndMeth=Floor
  Degrees to Radians{1..5} (5 alike) : simulink_extras/Transformations/Degrees to Radians
  Delay : Delay  DelayLength=1  InitialConditionSource=Input port
      settings: InputPortMap=u0,p4
  Delay1 : Delay  DelayLength=1  InitialConditionSource=Input port
      settings: InputPortMap=u0,p4
  Demux : Demux  Outputs=6
  Demux{4..5,7..8,11} (5 alike) : Demux  Outputs=3
  GPSflagcheck : MATLAB Function  TreatAsAtomicUnit=on
  Gain : Gain  Gain=-1
  Matrix Multiply1 : Product  Multiplication=Matrix(*)
  MesurementUpdate : MATLAB Function  TreatAsAtomicUnit=on
  MesurementValid : MATLAB Function  TreatAsAtomicUnit=on
  Mux{,2..5} (5 alike) : Mux  Inputs=3
  Mux6 : Mux  Inputs=5
  Rmat_DTNS_GPS_ori : Constant  Value=diag([ (6.6/sqrt(25))^2 (6.6/sqrt(25))^2 (1/sqrt(25))^2 (0.5/sqrt(25))^2 (0.5/sqrt(25))^2 (0.5/sqrt(25))^2 ]);
  Rmat_DTNS_TRN : Constant  Value=diag((35/sqrt(25))^2);
  Rotation Angles to Direction Cosine Matrix : sharedtransform/Rotation Angles to Direction Cosine Matrix  rotationOrder=ZYX  aMode=aMode
      settings: SourceProductBaseCode=AE,PW,DR,MT,VE
  Selector : Selector  InputPortWidth=3  IndexOptions=Index vector (dialog)  Indices=[3 2 1]  OutputSizes=1
  Terminator : Terminator
  Terminator1 : Terminator
  Terminator7 : Terminator
  Transpose : Math  Operator=transpose  SignedPower=on
  residualValidCheck2 : Subsystem
  Hmat_TRN : Outport
  zmat_TRN : Outport  Port=2
  Rmat_TRN : Outport  Port=3
  Hmat_GPS : Outport  Port=4
  zmat_GPS : Outport  Port=5  PortDimensions=[6 1]
  Rmat_GPS : Outport  Port=6
  GPSflag : Outport  Port=7
  wires:
  GPSflagcheck/1(GPSflag) -> [GPSflag], GPSflag/1
  Bus Selector3/2 -> Data Type Conversion/1  "<GPSEstHorErr>"
  Bus Selector3/6 -> GPSflagcheck/6(AccY)  "<AccelerationY>"
  Bus Selector3/4 -> GPSflagcheck/4(state)  "<GPS_State>"
  Bus Selector3/5 -> GPSflagcheck/5(GPSDataNotValid)  "<GPSDataNotValid>"
  Data Type Conversion/1 -> GPSflagcheck/2(EstHorErr)
  Bus Selector3/1 -> GPSflagcheck/1(FoM)  "<FigureofMerit>"
  Data Type Conversion1/1 -> GPSflagcheck/3(EstVerErr)
  Bus Selector3/3 -> Data Type Conversion1/1  "<GPSEstVerticalErr>"
  Bus Selector1/9 -> Mux2/3  "<VelocityZ>"
  Bus Selector1/12 -> Degrees to Radians3/1  "<TrueHeading>"
  Bus Selector1/11 -> Degrees to Radians2/1  "<Pitch>"
  Bus Selector1/10 -> Degrees to Radians1/1  "<Roll>"
  Bus Selector1/14 -> Mux3/2  "<INSTimeTag>"
  Bus Selector1/7 -> Mux2/1  "<VelocityX>"
  Mux2/1 -> Matrix Multiply1/2
  Bus Selector1/8 -> Mux2/2  "<VelocityY>"
  Mux/1 -> [RPY], Selector/1
  Matrix Multiply1/1 -> [INS_velNED]
  Degrees to Radians2/1 -> Mux/2
  Rotation Angles to Direction Cosine Matrix/1 -> Transpose/1
  Degrees to Radians1/1 -> Mux/1
  In_TRNInput/1 -> Bus Selector2/1, Bus Selector1/1, Bus Selector3/1
  Selector/1 -> Rotation Angles to Direction Cosine Matrix/1
  Mux3/1 -> [timetag]
  Bus Selector1/13 -> Mux3/1  "<GPStimeValid>"
  Degrees to Radians3/1 -> Mux/3
  Bus Selector1/15 -> Mux3/3  "<RALTTimeTag>"
  Transpose/1 -> Matrix Multiply1/1
  Bus Selector1/4 -> Degrees to Radians4/1  "<Latitude_GPS>"
  Bus Selector1/5 -> Degrees to Radians5/1  "<Longitude_GPS>"
  Bus Selector1/6 -> Mux4/3  "<Altitude_GPS>"
  Mux4/1 -> [GPS_LLA]
  Degrees to Radians4/1 -> Mux4/1
  Degrees to Radians5/1 -> Mux4/2
  Bus Selector1/1 -> Mux5/1  "<VelocityNorth>"
  Bus Selector1/2 -> Mux5/2  "<VelocityEast>"
  Bus Selector1/3 -> Gain/1  "<VelocityUp>"
  Gain/1 -> Mux5/3
  Mux5/1 -> [GPS_velNED]
  Delay1/1 -> MesurementValid/11(GPStimeValid_temp)
  Demux11/3 -> MesurementUpdate/14(velD_INS)
  Demux/5 -> Mux6/4
  Demux8/3 -> MesurementUpdate/11(velD_GPS)
  Demux7/3 -> MesurementUpdate/8(Alt_GPS)
  M/1 -> MesurementUpdate/15(M)
  [timetag] -> Demux5/1
  Mux6/1 -> Terminator7/1
  Demux5/1 -> Delay1/2, MesurementValid/10(GPStimeValid), Delay1/1
  Demux5/2 -> Terminator1/1
  Bus Selector4/2 -> Demux/1  "<Result_Prev>"
  [RPY] -> Demux4/1
  MesurementUpdate/4(z_GPS) -> MesurementValid/12(zmat_inGPS)
  Demux/4 -> Mux6/3
  Demux4/2 -> MesurementValid/3(pitch)
  [GPSflag] -> MesurementValid/13(GPS_flag)
  Delay/1 -> MesurementValid/7(RALTTimeTag_temp)
  [GPS_velNED] -> Demux8/1
  Demux11/2 -> MesurementUpdate/13(velE_INS)
  Bus Selector2/2 -> MesurementValid/8(RLATvalid)  "<RALTValid>"
  [INS_velNED] -> Demux11/1
  MesurementUpdate/2(z_TRN) -> MesurementValid/5(zmat_inTRN)
  INS_Lat/1 -> MesurementUpdate/17(psi), MesurementUpdate/2(Lat_INS)
  Demux7/1 -> MesurementUpdate/6(Lat_GPS)
  Demux8/1 -> MesurementUpdate/9(velN_GPS)
  Demux5/3 -> Delay/2, Delay/1, MesurementValid/6(RALTTimeTag)
  Bus Selector2/1 -> Data Type Conversion4/1  "<GPSDataNotValid>"
  N/1 -> MesurementUpdate/16(N)
  Data Type Conversion4/1 -> MesurementUpdate/1(GPSDataNotValid), MesurementValid/1(GPSDataNotValid)
  MesurementUpdate/1(Hmatrix_TRN) -> Hmat_TRN/1
  Rmat_DTNS_TRN/1 -> Rmat_TRN/1
  Rmat_DTNS_GPS_ori/1 -> Rmat_GPS/1
  INS_Lon/1 -> MesurementUpdate/3(Lon_INS)
  Demux4/1 -> MesurementValid/2(roll)
  Bus Selector4/1 -> residualValidCheck2/1(TRNDatapump)  "<residual>"
  [GPS_LLA] -> Demux7/1
  Demux/6 -> Mux6/5
  Demux7/2 -> MesurementUpdate/7(Lon_GPS)
  Demux11/1 -> MesurementUpdate/12(velN_INS)
  AND/1 -> MesurementValid/4(updateValid)
  Demux8/2 -> MesurementUpdate/10(velE_GPS)
  Demux/3 -> Mux6/2
  Data Type Conversion3/1 -> AND/2
  INS_Alt/1 -> MesurementUpdate/4(Alt_INS)
  residualValidCheck2/1(residualValid) -> AND/1, MesurementValid/9(residualValid)
  MesurementUpdate/3(Hmatrix_GPS) -> Hmat_GPS/1
  Demux/1 -> Data Type Conversion3/1
  Demux/2 -> Mux6/1
  Demux4/3 -> Terminator/1
  Bus Selector2/3 -> MesurementUpdate/5(RALTAltitude)  "<RALTAltitude>"
  MesurementValid/2(z_GPS) -> zmat_GPS/1
  MesurementValid/1(z_TRN) -> zmat_TRN/1
  In_TRNDatapump/1 -> Bus Selector4/1

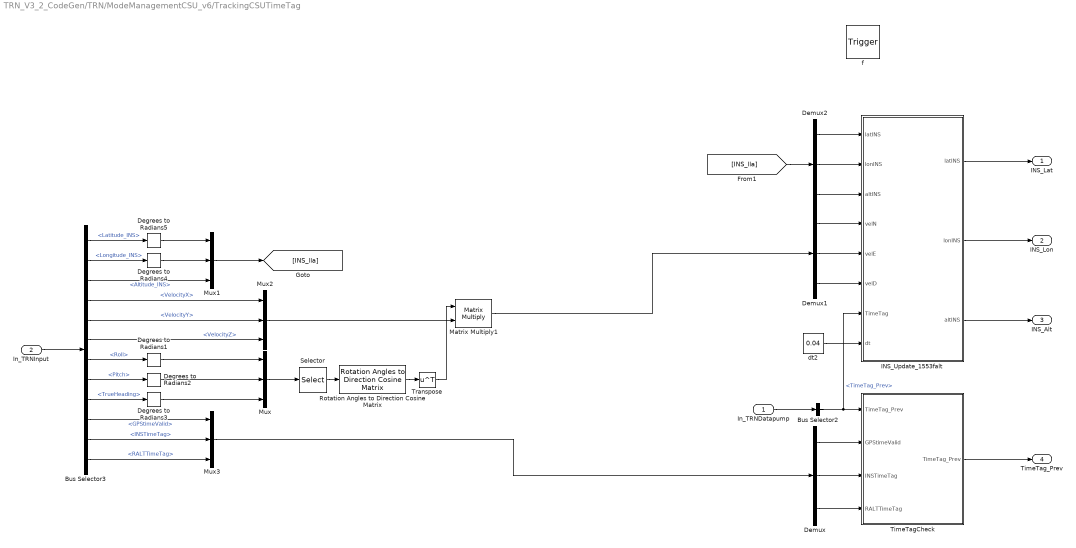
== system TRN_V3_2_CodeGen/TRN/ModeManagementCSU_v6/TrackingCSUTimeTag ==
  In_TRNDatapump : Inport  OutDataTypeStr=Bus: TRNDatapump  PortDimensions=1
  In_TRNInput : Inport  Port=2  OutDataTypeStr=Bus: TRNInput  PortDimensions=1
  f : TriggerPort  TriggerType=function-call  VariantControl=Variant
      settings: CopyFcn=Stateflow.SLINSF.SimulinkMan.removeBlockPreDeleteFcn  PreDeleteFcn=Stateflow.SLINSF.SimulinkMan.unsafePredeleteFcn
  Bus Selector2 : BusSelector  OutputSignals=TimeTag_Prev
  Bus Selector3 : BusSelector  OutputSignals=Latitude_INS,Longitude_INS,Altitude_INS,VelocityX,VelocityY,VelocityZ,Roll,Pitch,TrueHeading,GPStimeValid,INSTimeTag,RALTTimeTag
  Degrees to Radians{1..5} (5 alike) : simulink_extras/Transformations/Degrees to Radians
  Demux : Demux  Outputs=3
  Demux1 : Demux  Outputs=3
  Demux2 : Demux  Outputs=3
  INS_Update_1553falt : MATLAB Function  TreatAsAtomicUnit=on
  Matrix Multiply1 : Product  Multiplication=Matrix(*)
  Mux{,1..3} (4 alike) : Mux  Inputs=3
  Rotation Angles to Direction Cosine Matrix : sharedtransform/Rotation Angles to Direction Cosine Matrix  rotationOrder=ZYX  aMode=aMode
      settings: SourceProductBaseCode=AE,PW,DR,MT,VE
  Selector : Selector  InputPortWidth=3  IndexOptions=Index vector (dialog)  Indices=[3 2 1]  OutputSizes=1
  TimeTagCheck : MATLAB Function  TreatAsAtomicUnit=on
  Transpose : Math  Operator=transpose  SignedPower=on
  dt2 : Constant  Value=0.04  OutDataTypeStr=double
  INS_Lat : Outport
  INS_Lon : Outport  Port=2
  INS_Alt : Outport  Port=3
  TimeTag_Prev : Outport  Port=4  OutDataTypeStr=uint32  PortDimensions=6
  wires:
  dt2/1 -> INS_Update_1553falt/8(dt)
  INS_Update_1553falt/3(altINS) -> INS_Alt/1
  INS_Update_1553falt/2(lonINS) -> INS_Lon/1
  Demux/3 -> TimeTagCheck/4(RALTTimeTag)
  In_TRNDatapump/1 -> Bus Selector2/1
  Demux/1 -> TimeTagCheck/2(GPStimeValid)
  Demux/2 -> TimeTagCheck/3(INSTimeTag)
  TimeTagCheck/1(TimeTag_Prev) -> TimeTag_Prev/1
  Demux2/1 -> INS_Update_1553falt/1("latINS ")
  Demux2/2 -> INS_Update_1553falt/2("lonINS ")
  Demux2/3 -> INS_Update_1553falt/3("altINS ")
  Demux1/1 -> INS_Update_1553falt/4(velN)
  Demux1/2 -> INS_Update_1553falt/5(velE)
  Demux1/3 -> INS_Update_1553falt/6(velD)
  Bus Selector2/1 -> INS_Update_1553falt/7(TimeTag), TimeTagCheck/1("TimeTag_Prev ")  "<TimeTag_Prev>"
  INS_Update_1553falt/1(latINS) -> INS_Lat/1
  In_TRNInput/1 -> Bus Selector3/1
  Transpose/1 -> Matrix Multiply1/1
  Degrees to Radians1/1 -> Mux/1
  Rotation Angles to Direction Cosine Matrix/1 -> Transpose/1
  Degrees to Radians2/1 -> Mux/2
  Mux/1 -> Selector/1
  Mux2/1 -> Matrix Multiply1/2
  Degrees to Radians3/1 -> Mux/3
  Bus Selector3/7 -> Degrees to Radians1/1  "<Roll>"
  Bus Selector3/6 -> Mux2/3  "<VelocityZ>"
  Bus Selector3/8 -> Degrees to Radians2/1  "<Pitch>"
  Bus Selector3/9 -> Degrees to Radians3/1  "<TrueHeading>"
  Bus Selector3/4 -> Mux2/1  "<VelocityX>"
  Bus Selector3/5 -> Mux2/2  "<VelocityY>"
  Selector/1 -> Rotation Angles to Direction Cosine Matrix/1
  Bus Selector3/1 -> Degrees to Radians5/1  "<Latitude_INS>"
  Bus Selector3/3 -> Mux1/3  "<Altitude_INS>"
  Bus Selector3/2 -> Degrees to Radians4/1  "<Longitude_INS>"
  Degrees to Radians5/1 -> Mux1/1
  Degrees to Radians4/1 -> Mux1/2
  Mux1/1 -> [INS_lla]
  Bus Selector3/11 -> Mux3/2  "<INSTimeTag>"
  Bus Selector3/10 -> Mux3/1  "<GPStimeValid>"
  Bus Selector3/12 -> Mux3/3  "<RALTTimeTag>"
  Mux3/1 -> Demux/1
  Matrix Multiply1/1 -> Demux1/1
  [INS_lla] -> Demux2/1

== system TRN_V3_2_CodeGen/TRN/ModeManagementCSU_v6/ValidityCheck ==
  continuousValid : Inport  OutDataTypeStr=boolean  PortDimensions=1
  latINSErrTRN : Inport  Port=2  OutDataTypeStr=double  PortDimensions=1
  lonINSErrTRN : Inport  Port=3  OutDataTypeStr=double  PortDimensions=1
  altINSErrTRN : Inport  Port=4  OutDataTypeStr=double  PortDimensions=1
  f : TriggerPort  TriggerType=function-call  VariantControl=Variant
      settings: CopyFcn=Stateflow.SLINSF.SimulinkMan.removeBlockPreDeleteFcn  PreDeleteFcn=Stateflow.SLINSF.SimulinkMan.unsafePredeleteFcn
  Scope1 : Scope  NumInputPorts=2
  ValidityCheck function : MATLAB Function  TreatAsAtomicUnit=on
  TRNEstOfINSLatitudeErr : Outport  VectorParamsAs1DForOutWhenUnconnected=off
  TRNEstOfINSLongitudeErr : Outport  Port=2
  TRNEstOfINSAltitudeErr : Outport  Port=3
  AircraftPositionCorrectionValid : Outport  Port=4  OutDataTypeStr=boolean
  wires:
  ValidityCheck function/4(AircraftPositionCorrectionValid) -> AircraftPositionCorrectionValid/1
  continuousValid/1 -> Scope1/1, ValidityCheck function/1(continuousValid)
  latINSErrTRN/1 -> ValidityCheck function/2(latINSErrTRN)
  lonINSErrTRN/1 -> ValidityCheck function/3(lonINSErrTRN)
  altINSErrTRN/1 -> ValidityCheck function/4(altINSErrTRN)
  ValidityCheck function/3(TRNEstOfINSAltitudeErr) -> TRNEstOfINSAltitudeErr/1
  ValidityCheck function/2(TRNEstOfINSLongitudeErr) -> TRNEstOfINSLongitudeErr/1
  ValidityCheck function/1(TRNEstOfINSLatitudeErr) -> Scope1/2, TRNEstOfINSLatitudeErr/1

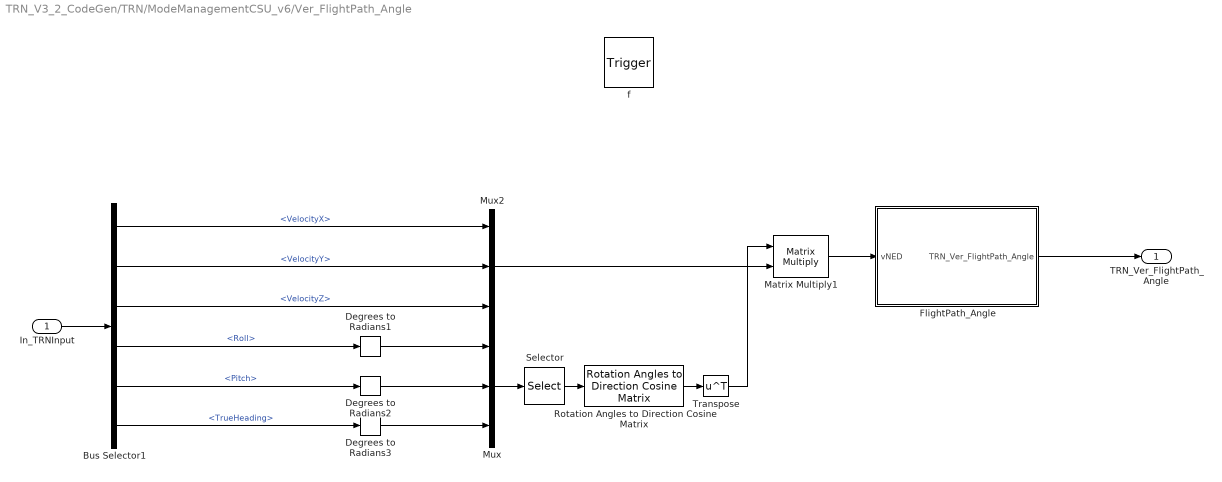
== system TRN_V3_2_CodeGen/TRN/ModeManagementCSU_v6/Ver_FlightPath_Angle ==
  In_TRNInput : Inport  OutDataTypeStr=Bus: TRNInput  PortDimensions=1
  f : TriggerPort  TriggerType=function-call  VariantControl=Variant
      settings: CopyFcn=Stateflow.SLINSF.SimulinkMan.removeBlockPreDeleteFcn  PreDeleteFcn=Stateflow.SLINSF.SimulinkMan.unsafePredeleteFcn
  Bus Selector1 : BusSelector  OutputSignals=VelocityX,VelocityY,VelocityZ,Roll,Pitch,TrueHeading
  Degrees to Radians1 : simulink_extras/Transformations/Degrees to Radians
  Degrees to Radians2 : simulink_extras/Transformations/Degrees to Radians
  Degrees to Radians3 : simulink_extras/Transformations/Degrees to Radians
  FlightPath_Angle : MATLAB Function  TreatAsAtomicUnit=on
  Matrix Multiply1 : Product  Multiplication=Matrix(*)
  Mux : Mux  Inputs=3
  Mux2 : Mux  Inputs=3
  Rotation Angles to Direction Cosine Matrix : sharedtransform/Rotation Angles to Direction Cosine Matrix  rotationOrder=ZYX  aMode=aMode
      settings: SourceProductBaseCode=AE,PW,DR,MT,VE
  Selector : Selector  InputPortWidth=3  IndexOptions=Index vector (dialog)  Indices=[3 2 1]  OutputSizes=1
  Transpose : Math  Operator=transpose  SignedPower=on
  TRN_Ver_FlightPath_Angle : Outport  OutDataTypeStr=double
  wires:
  Bus Selector1/4 -> Degrees to Radians1/1  "<Roll>"
  Transpose/1 -> Matrix Multiply1/1
  Selector/1 -> Rotation Angles to Direction Cosine Matrix/1
  FlightPath_Angle/1(TRN_Ver_FlightPath_Angle) -> TRN_Ver_FlightPath_Angle/1
  Degrees to Radians1/1 -> Mux/1
  Bus Selector1/1 -> Mux2/1  "<VelocityX>"
  In_TRNInput/1 -> Bus Selector1/1
  Bus Selector1/6 -> Degrees to Radians3/1  "<TrueHeading>"
  Mux2/1 -> Matrix Multiply1/2
  Degrees to Radians3/1 -> Mux/3
  Degrees to Radians2/1 -> Mux/2
  Bus Selector1/5 -> Degrees to Radians2/1  "<Pitch>"
  Bus Selector1/3 -> Mux2/3  "<VelocityZ>"
  Mux/1 -> Selector/1
  Matrix Multiply1/1 -> FlightPath_Angle/1(vNED)
  Rotation Angles to Direction Cosine Matrix/1 -> Transpose/1
  Bus Selector1/2 -> Mux2/2  "<VelocityY>"
